simulink model "PlanarRobot"  (R2017a)
settings: Solver=ode3  StartTime=0.0  StopTime=10.0  FixedStep=0.01  RelTol=1e-3  EnableMultiTasking=on
settings Model: Creator=ejlobato  LastModifiedBy=Henry
settings DataIOCC: LimitDataPoints=on  SaveFormat=Array
settings OptimizationCC: LifeSpan=inf
settings DebuggingCC: UnderspecifiedInitializationDetection=Classic  MergeDetectMultiDrivingBlocksExec=none  SolverPrmCheckMsg=warning  StateNameClashWarn=warning  SFUnexpectedBacktrackingDiag=warning  SFNoUnconditionalDefaultTransitionDiag=warning  SFExecutionAtInitializationDiag=none
settings HardwareCC: ProdBitPerPointer=32  ProdBitPerSizeT=32  ProdBitPerPtrDiffT=32  ProdLargestAtomicFloat=None  ProdIntDivRoundTo=Undefined  ProdEndianess=Unspecified  ProdWordSize=32  ProdHWDeviceType=32-bit Generic
settings ModelReferenceCC: PropagateSignalLabelsOutOfModel=off
settings GRTTargetCC: TargetLangStandard=C89/C90 (ANSI)  GeneratePreprocessorConditionals=Disable all
settings ConfigComp: CovMetricSettings=dw  CovHtmlReporting=on  CovSaveCumulativeToWorkspaceVar=on  CovSaveSingleToWorkspaceVar=on  CovExternalEMLEnable=off

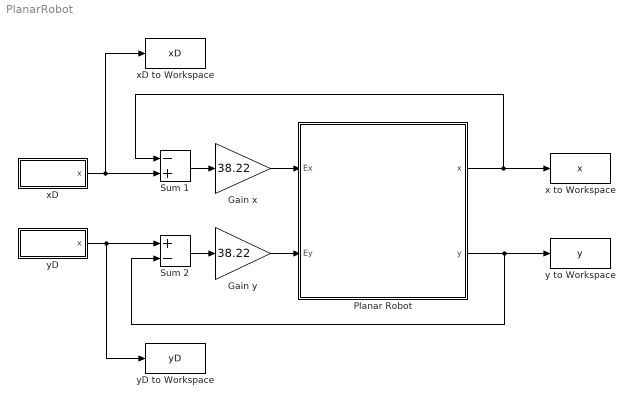
== system PlanarRobot ==
  Gain x : Gain  Gain=38.22
  Gain y : Gain  Gain=38.22
  Planar Robot : Subsystem
  Sum 1 : Sum  Inputs=-+
  Sum 2 : Sum  Inputs=+-
  x to Workspace : ToWorkspace  VariableName=x  SaveFormat=Timeseries  SampleTime=-1
  xD : Subsystem
  "xD to Workspace " : ToWorkspace  VariableName=xD  SaveFormat=Timeseries  SampleTime=-1
  y to Workspace : ToWorkspace  VariableName=y  SaveFormat=Timeseries  SampleTime=-1
  yD : Subsystem
  yD to Workspace : ToWorkspace  VariableName=yD  SaveFormat=Timeseries  SampleTime=-1
  wires:
  Planar Robot/2(y) -> Sum 2/2, y to Workspace/1
  xD/1(x) -> "xD to Workspace "/1, Sum 1/2
  Sum 1/1 -> Gain x/1
  Planar Robot/1(x) -> Sum 1/1, x to Workspace/1
  Sum 2/1 -> Gain y/1
  yD/1(x) -> yD to Workspace/1, Sum 2/1
  Gain x/1 -> Planar Robot/1(Ex)
  Gain y/1 -> Planar Robot/2(Ey)

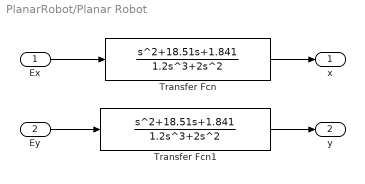
== system PlanarRobot/Planar Robot ==
  Ex : Inport
  Ey : Inport  Port=2
  Transfer Fcn : TransferFcn  Numerator=[1 18.51 1.841]  Denominator=[1.2 2 0 0]
  Transfer Fcn1 : TransferFcn  Numerator=[1 18.51 1.841]  Denominator=[1.2 2 0 0]
  x : Outport
  y : Outport  Port=2
  wires:
  Ex/1 -> Transfer Fcn/1
  Transfer Fcn/1 -> x/1
  Ey/1 -> Transfer Fcn1/1
  Transfer Fcn1/1 -> y/1

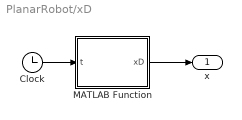
== system PlanarRobot/xD ==
  Clock : Clock
  MATLAB Function : MATLAB Function  TreatAsAtomicUnit=on
  x : Outport
  wires:
  MATLAB Function/1(xD) -> x/1
  Clock/1 -> MATLAB Function/1(t)

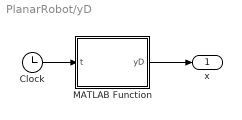
== system PlanarRobot/yD ==
  Clock : Clock
  MATLAB Function : MATLAB Function  TreatAsAtomicUnit=on
  x : Outport
  wires:
  MATLAB Function/1(yD) -> x/1
  Clock/1 -> MATLAB Function/1(t)

== matlab function PlanarRobot/xD/MATLAB Function ==
  data: xD output; t input
function xD = fcn(t)
% x-coordinates of desired trajectory.

xD = -t.*(t>=0).*(t<0.5) + ...
   -0.5*(t>=0.5).*(t<1.5) + ...
   (t-2).*(t>=1.5).*(t<2.5) + ...
   0.5*(t>=2.5).*(t<3.5) + ...
   -(t-4).*(t>=3.5).*(t<4) + ...
   -0.5*sin(2*(t-4)).*(t>=4).*(t<4+pi);

== matlab function PlanarRobot/yD/MATLAB Function ==
  data: yD output; t input
function yD = fcn(t)
% y-coordinates of desired trajectory.

yD = 0*(t>=0).*(t<0.5) + ...
    (t-0.5).*(t>=0.5).*(t<1.5) + ...
    1*(t>=1.5).*(t<2.5) + ...
    -(t-3.5).*(t>=2.5).*(t<3.5) + ...
    0*(t>=3.5).*(t<4) + ...
    -0.5*(cos(2*(t-4))-1).*(t>=4).*(t<4+pi);
